simulink model "online_diary"  (R2025a)
settings: Solver=VariableStepAuto  StartTime=0.0  StopTime=10.0  RelTol=1e-3
settings Model: Creator=Admin  LastModifiedBy=Admin

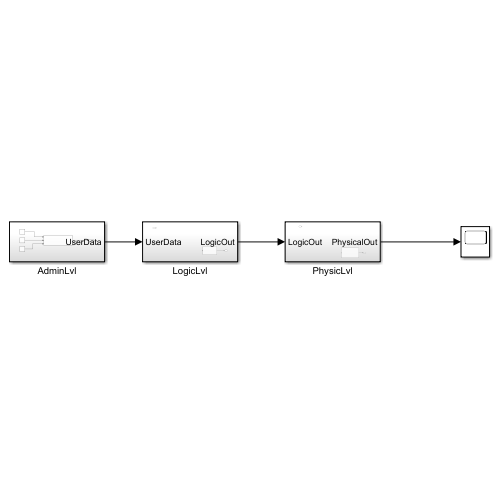
[thumbnail: Simulink's stored preview of the top-level diagram]
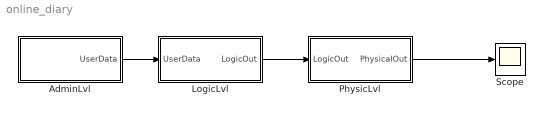
== system online_diary ==
  AdminLvl : Subsystem
  LogicLvl : Subsystem
  PhysicLvl : Subsystem
  Scope : Scope
      settings: ActiveDisplayYMinimum=-1  ActiveDisplayYMaximum=1
  wires:
  AdminLvl/1(UserData) -> LogicLvl/1(UserData)
  LogicLvl/1(LogicOut) -> PhysicLvl/1(LogicOut)
  PhysicLvl/1(PhysicalOut) -> Scope/1

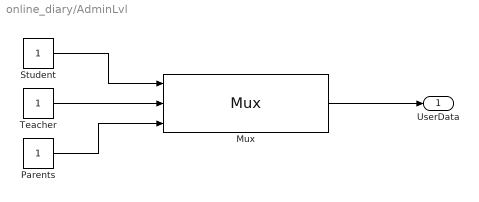
== system online_diary/AdminLvl ==
  Mux : Mux  Inputs=3
  Parents : Constant
  Student : Constant
  Teacher : Constant
  UserData : Outport
  wires:
  Student/1 -> Mux/1
  Teacher/1 -> Mux/2
  Parents/1 -> Mux/3
  Mux/1 -> UserData/1

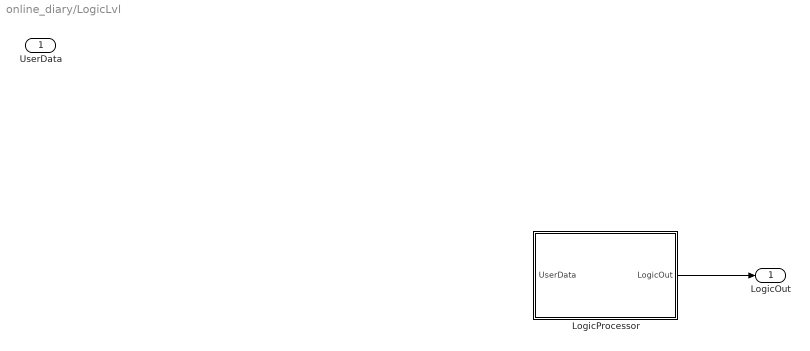
== system online_diary/LogicLvl ==
  UserData : Inport
  LogicProcessor : MATLAB Function  TreatAsAtomicUnit=on
  LogicOut : Outport
  wires:
  LogicProcessor/1(LogicOut) -> LogicOut/1

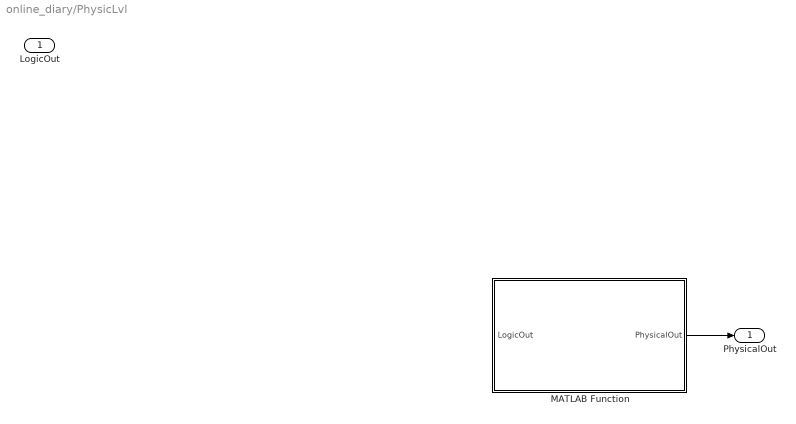
== system online_diary/PhysicLvl ==
  LogicOut : Inport
  MATLAB Function : MATLAB Function  TreatAsAtomicUnit=on
  PhysicalOut : Outport
  wires:
  MATLAB Function/1(PhysicalOut) -> PhysicalOut/1

== matlab function online_diary/PhysicLvl/MATLAB Function ==
  data: LogicOut input; PhysicalOut output
function PhysicalOut = PhysicalLayer(LogicOut)
% Фізичний рівень: передача даних між клієнтом, сервером і БД

% Явно визначаємо тип і розмір виходу
PhysicalOut = zeros(1,1); % одиничне число

if LogicOut == 1
    disp('Дані передані до сервера і збережені в базі даних.');
    PhysicalOut = 1;
else
    disp('Немає даних для збереження.');
    PhysicalOut = 0;
end
end

== matlab function online_diary/LogicLvl/LogicProcessor ==
  data: UserData input; LogicOut output
function LogicOut = LogicProcessor(UserData)

LogicOut = zeros(1,1); 

if any(UserData > 0)
    disp('Обробка даних: оновлення оцінок, журналу, сповіщень...');
    LogicOut = 1;
else
    disp('Дані відсутні.');
    LogicOut = 0;
end
end
